simulink model "hvac_heat_pump"  (R2024a)
settings: Solver=VariableStepAuto  StartTime=0.0  StopTime=30000  RelTol=1e-3
settings Model: Creator=ml4  LastModifiedBy=ml4

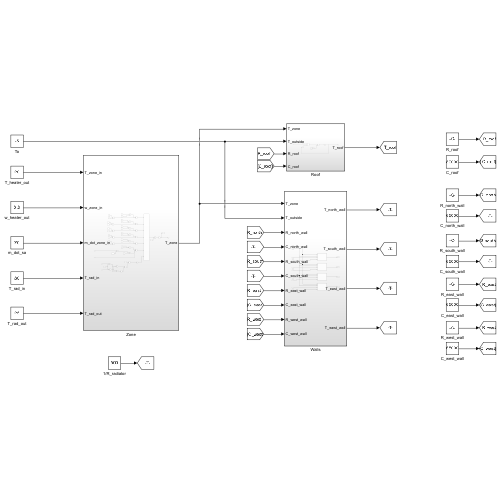
[thumbnail: Simulink's stored preview of the top-level diagram]
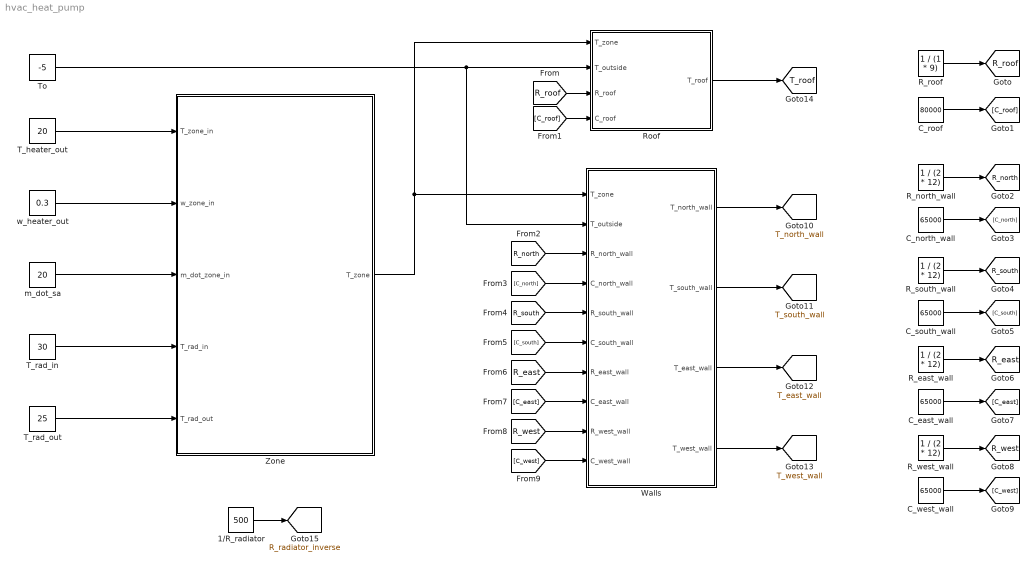
== system hvac_heat_pump ==
  1/R_radiator : Constant  Value=500
  C_east_wall : Constant  Value=65000
  C_north_wall : Constant  Value=65000
  C_roof : Constant  Value=80000
  C_south_wall : Constant  Value=65000
  C_west_wall : Constant  Value=65000
  R_east_wall : Constant  Value=1 / (2 * 12)
  R_north_wall : Constant  Value=1 / (2 * 12)
  R_roof : Constant  Value=1 / (1 * 9)
  R_south_wall : Constant  Value=1 / (2 * 12)
  R_west_wall : Constant  Value=1 / (2 * 12)
  Roof : Subsystem
  T_heater_out : Constant  Value=20
  T_rad_in : Constant  Value=30
  T_rad_out : Constant  Value=25
  To : Constant  Value=-5
  Walls : Subsystem
  Zone : Subsystem
  m_dot_sa : Constant  Value=20
  w_heater_out : Constant  Value=0.3
  tag scope: R_east=global, R_north=global, R_radiator_inverse=global, R_roof=global, R_south=global, R_west=global, T_east_wall=global, T_north_wall=global, T_roof=global, T_south_wall=global, T_west_wall=global
  wires:
  To/1 -> Walls/2(T_outside), Roof/2(T_outside)
  R_roof/1 -> [R_roof]
  [R_roof] -> Roof/3(R_roof)
  C_roof/1 -> [C_roof]
  [C_roof] -> Roof/4(C_roof)
  R_north_wall/1 -> [R_north]
  C_north_wall/1 -> [C_north]
  R_south_wall/1 -> [R_south]
  C_south_wall/1 -> [C_south]
  R_east_wall/1 -> [R_east]
  C_east_wall/1 -> [C_east]
  R_west_wall/1 -> [R_west]
  C_west_wall/1 -> [C_west]
  [R_north] -> Walls/3(R_north_wall)
  [C_north] -> Walls/4(C_north_wall)
  [R_south] -> Walls/5(R_south_wall)
  [C_south] -> Walls/6(C_south_wall)
  [R_east] -> Walls/7(R_east_wall)
  [C_east] -> Walls/8(C_east_wall)
  [R_west] -> Walls/9(R_west_wall)
  [C_west] -> Walls/10(C_west_wall)
  Walls/1(T_north_wall) -> [T_north_wall]
  Walls/2(T_south_wall) -> [T_south_wall]
  Walls/3(T_east_wall) -> [T_east_wall]
  Walls/4(T_west_wall) -> [T_west_wall]
  Roof/1(T_roof) -> [T_roof]
  Zone/1(T_zone) -> Roof/1(T_zone), Walls/1(T_zone)
  T_heater_out/1 -> Zone/1(T_zone_in)
  w_heater_out/1 -> Zone/2(w_zone_in)
  m_dot_sa/1 -> Zone/3(m_dot_zone_in)
  T_rad_in/1 -> Zone/4(T_rad_in)
  T_rad_out/1 -> Zone/5(T_rad_out)
  1/R_radiator/1 -> [R_radiator_inverse]

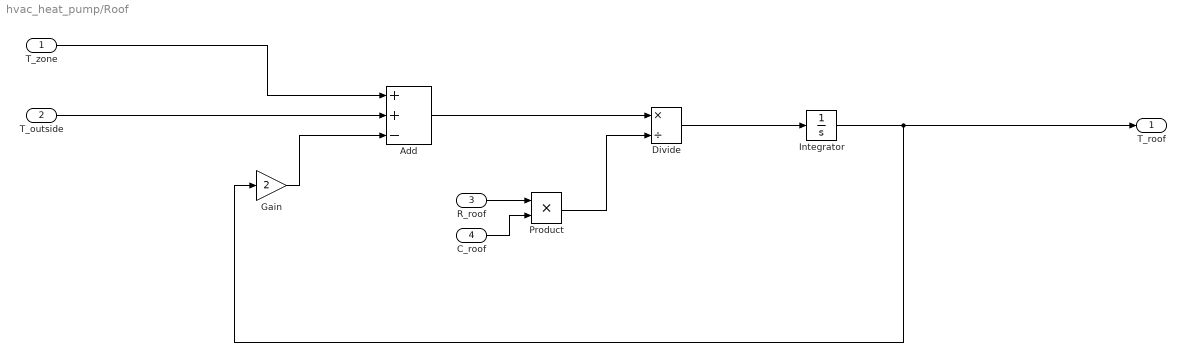
== system hvac_heat_pump/Roof ==
  T_zone : Inport
  T_outside : Inport  Port=2
  R_roof : Inport  Port=3
  C_roof : Inport  Port=4
  Add : Sum  Inputs=++-
  Divide : Product  Inputs=*/
  Gain : Gain  Gain=2
  Integrator : Integrator
  Product : Product
  T_roof : Outport
  wires:
  T_zone/1 -> Add/1
  Integrator/1 -> T_roof/1, Gain/1
  Product/1 -> Divide/2
  Gain/1 -> Add/3
  Divide/1 -> Integrator/1
  Add/1 -> Divide/1
  T_outside/1 -> Add/2
  R_roof/1 -> Product/1
  C_roof/1 -> Product/2

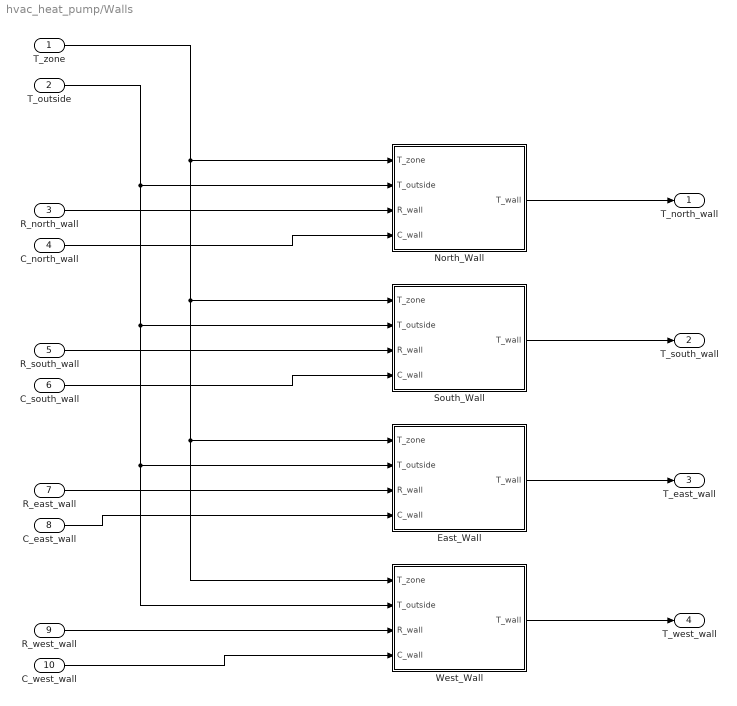
== system hvac_heat_pump/Walls ==
  T_zone : Inport
  T_outside : Inport  Port=2
  R_north_wall : Inport  Port=3
  C_north_wall : Inport  Port=4
  R_south_wall : Inport  Port=5
  C_south_wall : Inport  Port=6
  R_east_wall : Inport  Port=7
  C_east_wall : Inport  Port=8
  R_west_wall : Inport  Port=9
  C_west_wall : Inport  Port=10
  East_Wall : Subsystem
  North_Wall : Subsystem
  South_Wall : Subsystem
  West_Wall : Subsystem
  T_north_wall : Outport
  T_south_wall : Outport  Port=2
  T_east_wall : Outport  Port=3
  T_west_wall : Outport  Port=4
  wires:
  T_outside/1 -> North_Wall/2(T_outside), South_Wall/2(T_outside), East_Wall/2(T_outside), West_Wall/2(T_outside)
  T_zone/1 -> North_Wall/1(T_zone), South_Wall/1(T_zone), East_Wall/1(T_zone), West_Wall/1(T_zone)
  West_Wall/1(T_wall) -> T_west_wall/1
  South_Wall/1(T_wall) -> T_south_wall/1
  East_Wall/1(T_wall) -> T_east_wall/1
  North_Wall/1(T_wall) -> T_north_wall/1
  R_north_wall/1 -> North_Wall/3(R_wall)
  C_north_wall/1 -> North_Wall/4(C_wall)
  R_south_wall/1 -> South_Wall/3(R_wall)
  C_south_wall/1 -> South_Wall/4(C_wall)
  R_east_wall/1 -> East_Wall/3(R_wall)
  C_east_wall/1 -> East_Wall/4(C_wall)
  R_west_wall/1 -> West_Wall/3(R_wall)
  C_west_wall/1 -> West_Wall/4(C_wall)

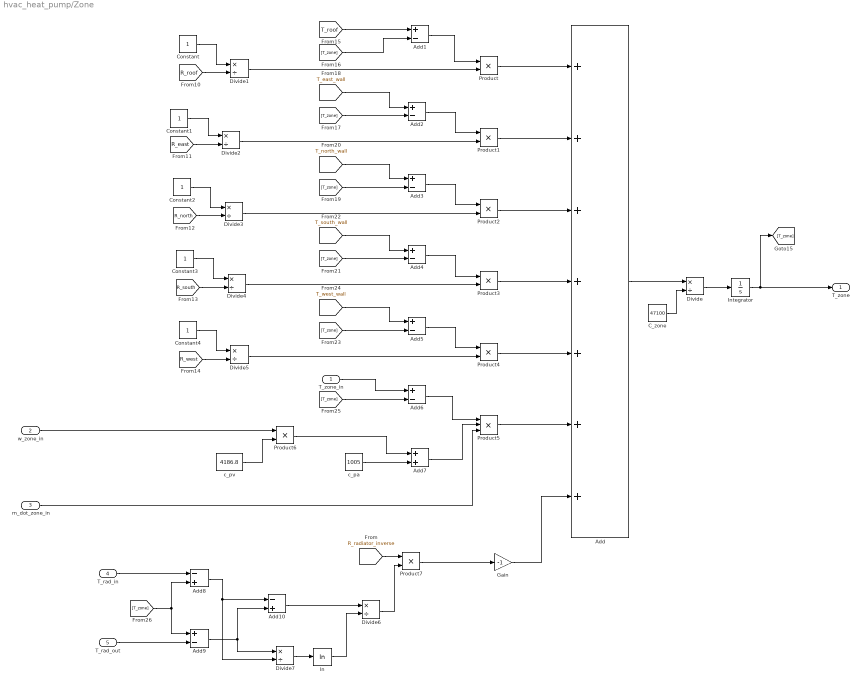
== system hvac_heat_pump/Zone ==
  T_zone_in : Inport
  w_zone_in : Inport  Port=2
  m_dot_zone_in : Inport  Port=3
  T_rad_in : Inport  Port=4
  T_rad_out : Inport  Port=5
  Add : Sum  Inputs=+++++++
  Add{1..6,9} (7 alike) : Sum  Inputs=+-
  Add10 : Sum  Inputs=-+
  Add7 : Sum
  Add8 : Sum  Inputs=-+
  C_zone : Constant  Value=47100
  Constant{,1..4} (5 alike) : Constant
  Divide{,1..7} (8 alike) : Product  Inputs=*/
  Gain : Gain  Gain=-1
  Integrator : Integrator
  Product{,1..4,6..7} (7 alike) : Product
  Product5 : Product  Inputs=3
  c_pa : Constant  Value=1005
  c_pv : Constant  Value=4186.8
  ln : Math  Operator=log
  T_zone : Outport
  wires:
  Product2/1 -> Add/3
  Divide3/1 -> Product2/2
  Add/1 -> Divide/1
  [R_roof] -> Divide1/2
  T_rad_in/1 -> Add8/1
  C_zone/1 -> Divide/2
  [T_east_wall] -> Add2/1
  Add9/1 -> Divide7/1, Add10/2
  Constant3/1 -> Divide4/1
  [T_zone] -> Add2/2
  Integrator/1 -> T_zone/1, [T_zone]
  T_rad_out/1 -> Add9/2
  [R_east] -> Divide2/2
  Gain/1 -> Add/7
  c_pv/1 -> Product6/2
  Product7/1 -> Gain/1
  c_pa/1 -> Add7/2
  Constant2/1 -> Divide3/1
  Constant1/1 -> Divide2/1
  Constant/1 -> Divide1/1
  Product6/1 -> Add7/1
  Product1/1 -> Add/2
  [T_south_wall] -> Add4/1
  [R_south] -> Divide4/2
  Add7/1 -> Product5/2
  [T_zone] -> Add1/2
  [T_zone] -> Add6/2
  Divide7/1 -> ln/1
  Product3/1 -> Add/4
  Divide2/1 -> Product1/2
  Add4/1 -> Product3/1
  Divide/1 -> Integrator/1
  Product/1 -> Add/1
  [T_west_wall] -> Add5/1
  T_zone_in/1 -> Add6/1
  [T_north_wall] -> Add3/1
  [R_north] -> Divide3/2
  w_zone_in/1 -> Product6/1
  Add1/1 -> Product/1
  [T_roof] -> Add1/1
  Divide6/1 -> Product7/2
  Divide1/1 -> Product/2
  Product5/1 -> Add/6
  Add10/1 -> Divide6/1
  [T_zone] -> Add3/2
  Constant4/1 -> Divide5/1
  [T_zone] -> Add4/2
  Add8/1 -> Divide7/2, Add10/1
  Add2/1 -> Product1/1
  [T_zone] -> Add9/1, Add8/2
  [T_zone] -> Add5/2
  Divide5/1 -> Product4/2
  Add3/1 -> Product2/1
  Add5/1 -> Product4/1
  Divide4/1 -> Product3/2
  m_dot_zone_in/1 -> Product5/3
  Add6/1 -> Product5/1
  [R_west] -> Divide5/2
  Product4/1 -> Add/5
  ln/1 -> Divide6/2
  [R_radiator_inverse] -> Product7/1

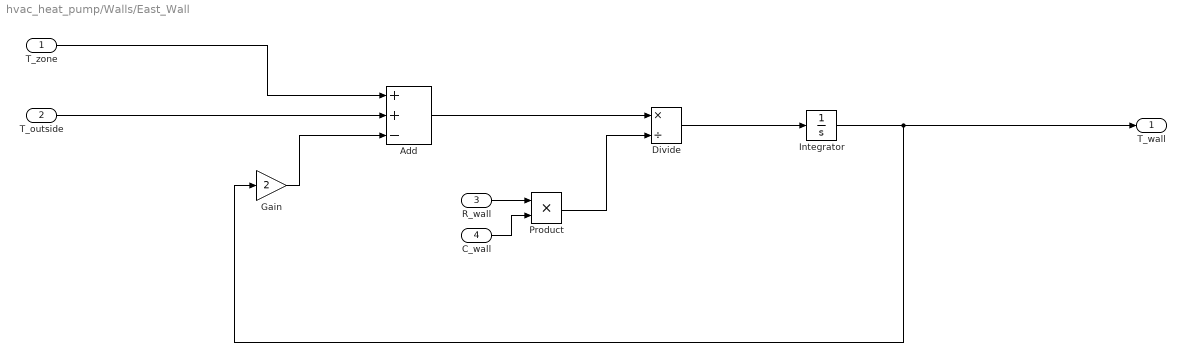
== system hvac_heat_pump/Walls/East_Wall ==
  T_zone : Inport
  T_outside : Inport  Port=2
  R_wall : Inport  Port=3
  C_wall : Inport  Port=4
  Add : Sum  Inputs=++-
  Divide : Product  Inputs=*/
  Gain : Gain  Gain=2
  Integrator : Integrator
  Product : Product
  T_wall : Outport
  wires:
  T_outside/1 -> Add/2
  Add/1 -> Divide/1
  Divide/1 -> Integrator/1
  Gain/1 -> Add/3
  Product/1 -> Divide/2
  Integrator/1 -> Gain/1, T_wall/1
  T_zone/1 -> Add/1
  R_wall/1 -> Product/1
  C_wall/1 -> Product/2

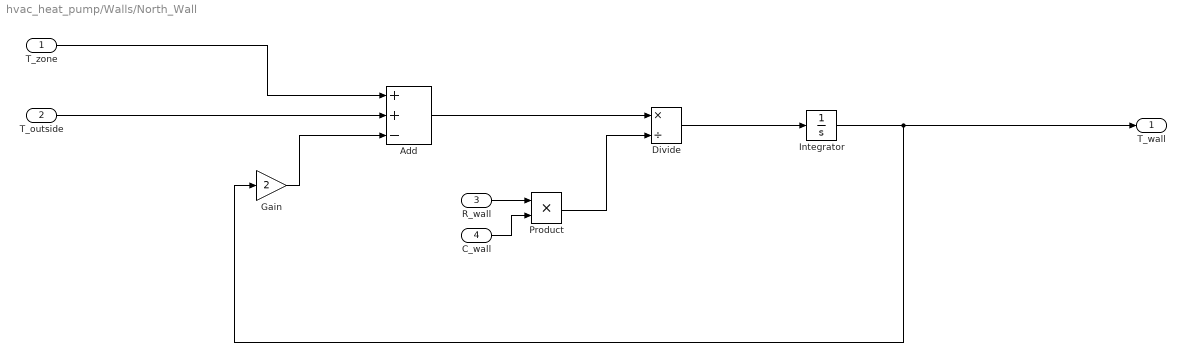
== system hvac_heat_pump/Walls/North_Wall ==
  T_zone : Inport
  T_outside : Inport  Port=2
  R_wall : Inport  Port=3
  C_wall : Inport  Port=4
  Add : Sum  Inputs=++-
  Divide : Product  Inputs=*/
  Gain : Gain  Gain=2
  Integrator : Integrator
  Product : Product
  T_wall : Outport
  wires:
  T_outside/1 -> Add/2
  Add/1 -> Divide/1
  Divide/1 -> Integrator/1
  Gain/1 -> Add/3
  Product/1 -> Divide/2
  Integrator/1 -> Gain/1, T_wall/1
  T_zone/1 -> Add/1
  R_wall/1 -> Product/1
  C_wall/1 -> Product/2

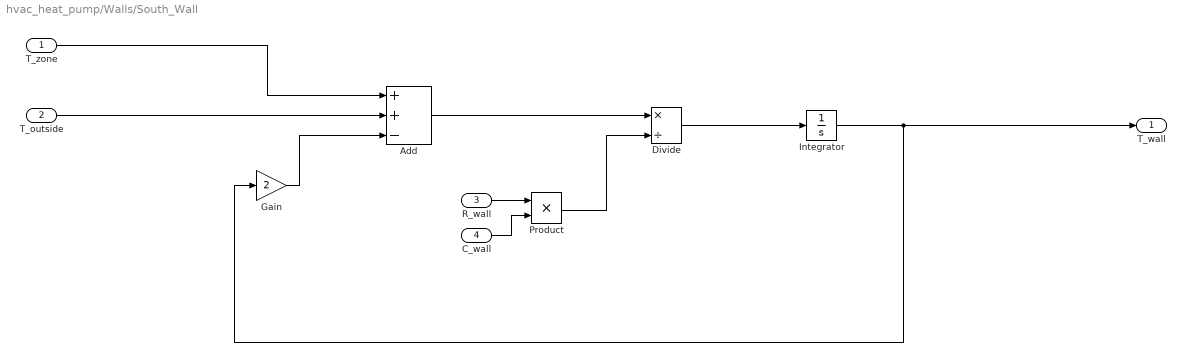
== system hvac_heat_pump/Walls/South_Wall ==
  T_zone : Inport
  T_outside : Inport  Port=2
  R_wall : Inport  Port=3
  C_wall : Inport  Port=4
  Add : Sum  Inputs=++-
  Divide : Product  Inputs=*/
  Gain : Gain  Gain=2
  Integrator : Integrator
  Product : Product
  T_wall : Outport
  wires:
  C_wall/1 -> Product/2
  R_wall/1 -> Product/1
  T_zone/1 -> Add/1
  Integrator/1 -> T_wall/1, Gain/1
  Product/1 -> Divide/2
  Gain/1 -> Add/3
  Divide/1 -> Integrator/1
  Add/1 -> Divide/1
  T_outside/1 -> Add/2

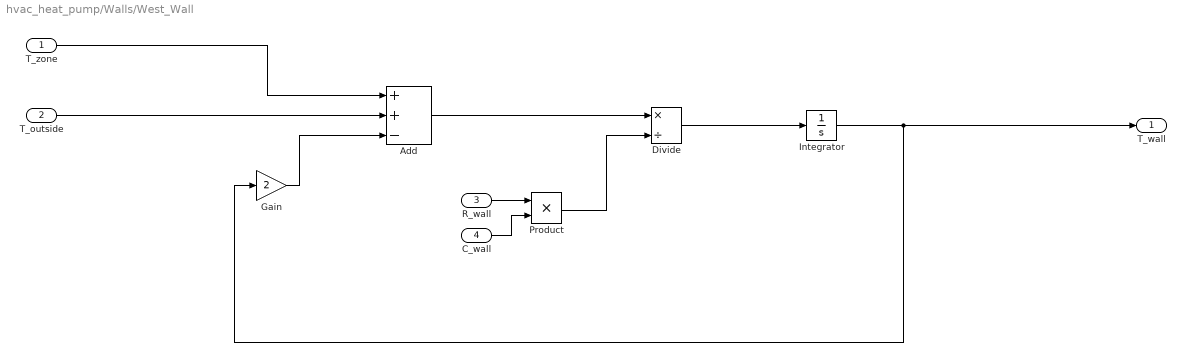
== system hvac_heat_pump/Walls/West_Wall ==
  T_zone : Inport
  T_outside : Inport  Port=2
  R_wall : Inport  Port=3
  C_wall : Inport  Port=4
  Add : Sum  Inputs=++-
  Divide : Product  Inputs=*/
  Gain : Gain  Gain=2
  Integrator : Integrator
  Product : Product
  T_wall : Outport
  wires:
  C_wall/1 -> Product/2
  R_wall/1 -> Product/1
  T_zone/1 -> Add/1
  Integrator/1 -> T_wall/1, Gain/1
  Product/1 -> Divide/2
  Gain/1 -> Add/3
  Divide/1 -> Integrator/1
  Add/1 -> Divide/1
  T_outside/1 -> Add/2
